simulink model "MainDrive_Kuehlung_V3_D"  (Simulink 7.6)
settings: Solver=ode45  StartTime=0.0  StopTime=SimulTime  RelTol=1e-3
values from neighbouring files (symbols this model uses):
  n = 0.8    [ParamtersSpindel_D.m]    (also in PlottingSpindel_Kuehlung_D.m = Scp_MainDrive.signals(4).values(:,1))
  n1 = 0.78    [ParamtersSpindel_D.m]
  n2 = 0.7    [ParamtersSpindel_D.m]
  p = 500    [ParamtersSpindel_D.m]
  p1 = 380    [ParamtersSpindel_D.m]
  p2 = 1100    [ParamtersSpindel_D.m]
  R = 25    [ParamtersSpindel_D.m]    (also in PlottingSpindel_Kuehlung_D.m = Scp_MainDriveT.signals(3).values(:,1)/1000)
  sb = 5.67*(10^-8)    (= 5.67e-08)    [ParamtersSpindel_D.m]
  T_amb = 290    [ParamtersSpindel_D.m]
  Venti_n2 = 273+40    (= 313)    [ParamtersSpindel_D.m]
undefined symbols (not defined in the file or in its folder): Job, magnitude, MainDrive, MainDriveCooling
libraries: simulink x1
settings Model: Creator=Coni  LastModifiedBy=conid

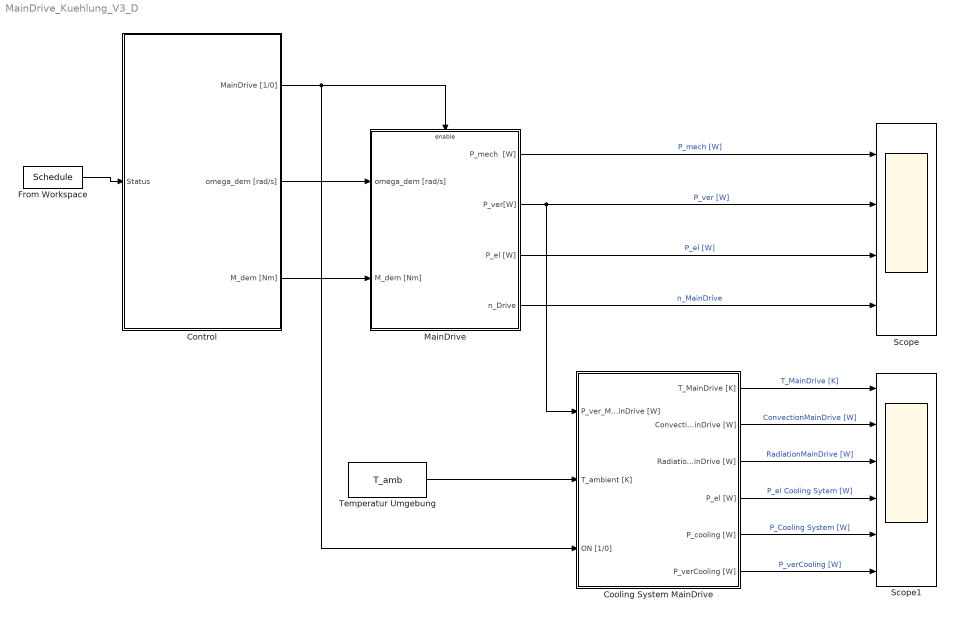
== system MainDrive_Kuehlung_V3_D ==
  Control : Subsystem  TreatAsAtomicUnit=on  mask{MainDrive=[0 1 1 1 1], Job=Job}
      mask prompts: Job "Job Struct"
      mask help:
      | Controls the components of the machine:
      |
      | Status:
      |     0. Off
      |     1. Standby
      |     2. Warmup
      |     3. Setting
      |     4. Machining
      |
      | If the status is machining, the job defined as
      |     - Job.time
      |     - Job.omega_dem
      |     - Job.M_dem
      | will be runned, and repeated.
      mask TabNameString: Status,Job
  Cooling System MainDrive : Subsystem  TreatAsAtomicUnit=on
  From Workspace : FromWorkspace  VariableName=Schedule  SampleTime=0  Interpolate=off  OutputAfterFinalValue=Holding final value
  MainDrive : Subsystem  TreatAsAtomicUnit=on
  Scope : Scope  NumInputPorts=4
      settings: TickLabels=on  TimeRange=100  YMin=0~-6e-010~-6e-010~-1.16573e-016  YMax=7e-026~-0~-0~-1.05471e-016  SaveName=Scp_MainDrive
  Scope1 : Scope  NumInputPorts=6
      settings: TickLabels=on  TimeRange=100  YMin=0~-5000~-2000~-0.1~-5~-5  YMax=16000~30000~14000~0.9~5~5  SaveName=Scp_MainDriveT
  Temperatur Umgebung : Constant  Value=T_amb
  wires:
  MainDrive/1(P_mech  [W]) -> Scope/1  "P_mech [W]"
  MainDrive/2(P_ver[W]) -> Scope/2, Cooling System MainDrive/1(P_ver_MainDrive [W])  "P_ver [W]"
  MainDrive/4(n_Drive) -> Scope/4  "n_MainDrive"
  Temperatur Umgebung/1 -> Cooling System MainDrive/2(T_ambient [K])
  MainDrive/3(P_el [W]) -> Scope/3  "P_el [W]"
  Cooling System MainDrive/1(T_MainDrive [K]) -> Scope1/1  "T_MainDrive [K]"
  Cooling System MainDrive/2(ConvectionMainDrive [W]) -> Scope1/2  "ConvectionMainDrive [W]"
  Cooling System MainDrive/3(RadiationMainDrive [W]) -> Scope1/3  "RadiationMainDrive [W]"
  Cooling System MainDrive/4(P_el [W]) -> Scope1/4  "P_el Cooling Sytem [W]"
  Cooling System MainDrive/5(P_cooling [W]) -> Scope1/5  "P_Cooling System [W]"
  Control/3(M_dem [Nm]) -> MainDrive/2(M_dem [Nm])
  From Workspace/1 -> Control/1(Status)
  Control/2(omega_dem [rad/s]) -> MainDrive/1(omega_dem [rad/s])
  Control/1(MainDrive [1/0]) -> MainDrive/Enable, Cooling System MainDrive/3(ON [1/0])
  Cooling System MainDrive/6(P_verCooling [W]) -> Scope1/6  "P_verCooling [W]"

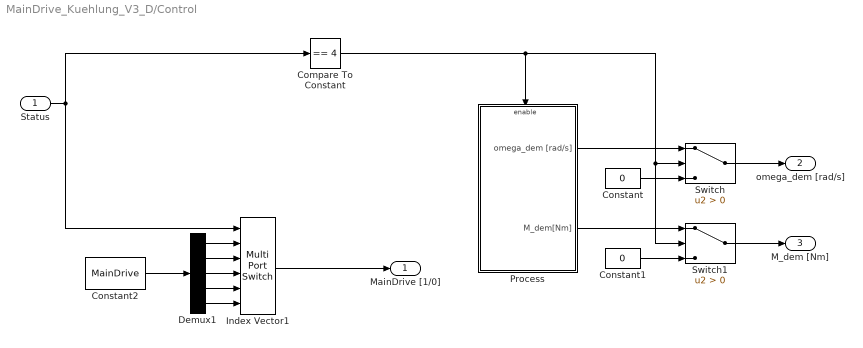
== system MainDrive_Kuehlung_V3_D/Control ==
  Status : Inport
  Compare To Constant : simulink/Logic and Bit Operations/Compare To Constant  SystemSampleTime=-1  relop===  const=4  LogicOutDataTypeMode=uint8
  Constant : Constant  Value=0
  Constant1 : Constant  Value=0
  Constant2 : Constant  Value=MainDrive
  Demux1 : Demux  Outputs=5
  Index Vector1 : MultiPortSwitch  DataPortOrder=Zero-based contiguous  Inputs=5  zeroidx=on
  Process : Subsystem  TreatAsAtomicUnit=on
  Switch : Switch  Criteria=u2 > Threshold
  Switch1 : Switch  Criteria=u2 > Threshold
  MainDrive [1/0] : Outport
  omega_dem [rad/s] : Outport  Port=2
  M_dem [Nm] : Outport  Port=3
  wires:
  Status/1 -> Compare To Constant/1, Index Vector1/1
  Demux1/1 -> Index Vector1/2
  Demux1/2 -> Index Vector1/3
  Demux1/3 -> Index Vector1/4
  Demux1/4 -> Index Vector1/5
  Demux1/5 -> Index Vector1/6
  Index Vector1/1 -> MainDrive [1/0]/1
  Compare To Constant/1 -> Process/Enable, Switch1/2, Switch/2
  Process/1(omega_dem [rad/s]) -> Switch/1
  Constant/1 -> Switch/3
  Process/2(M_dem[Nm]) -> Switch1/1
  Constant1/1 -> Switch1/3
  Switch/1 -> omega_dem [rad/s]/1
  Switch1/1 -> M_dem [Nm]/1
  Constant2/1 -> Demux1/1

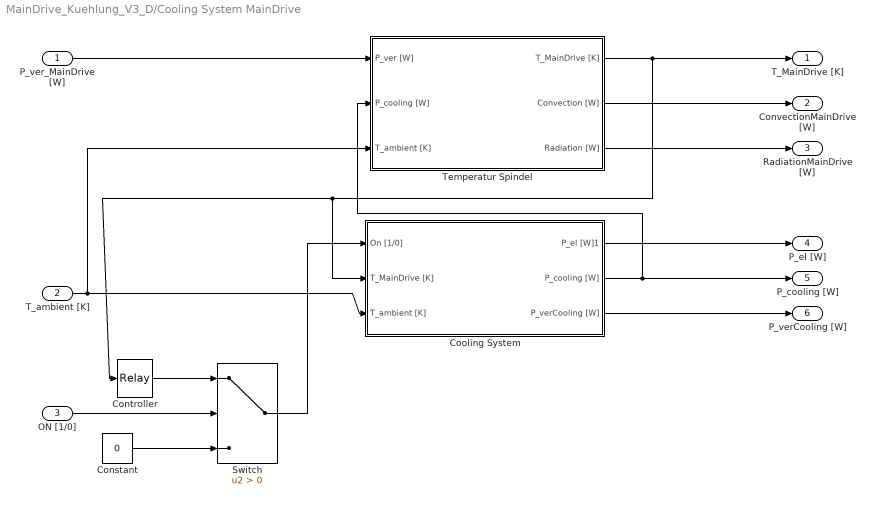
== system MainDrive_Kuehlung_V3_D/Cooling System MainDrive ==
  P_ver_MainDrive [W] : Inport
  T_ambient [K] : Inport  Port=2
  ON [1/0] : Inport  Port=3
  Constant : Constant  Value=0
  Controller : Relay  OnSwitchValue=MainDriveCooling.Tmax  OffSwitchValue=MainDriveCooling.Tmin
  Cooling System : Subsystem
  Switch : Switch  Criteria=u2 > Threshold
  Temperatur Spindel : Subsystem
  T_MainDrive [K] : Outport
  ConvectionMainDrive [W] : Outport  Port=2
  RadiationMainDrive [W] : Outport  Port=3
  P_el [W] : Outport  Port=4
  P_cooling [W] : Outport  Port=5
  P_verCooling [W] : Outport  Port=6
  wires:
  P_ver_MainDrive [W]/1 -> Temperatur Spindel/1(P_ver [W])
  Constant/1 -> Switch/3
  ON [1/0]/1 -> Switch/2
  Controller/1 -> Switch/1
  Temperatur Spindel/1(T_MainDrive [K]) -> Controller/1, Cooling System/2(T_MainDrive [K]), T_MainDrive [K]/1
  Switch/1 -> Cooling System/1(On [1/0])
  T_ambient [K]/1 -> Cooling System/3(T_ambient [K]), Temperatur Spindel/3(T_ambient [K])
  Temperatur Spindel/2(Convection [W]) -> ConvectionMainDrive [W]/1
  Temperatur Spindel/3(Radiation [W]) -> RadiationMainDrive [W]/1
  Cooling System/3(P_verCooling [W]) -> P_verCooling [W]/1
  Cooling System/1(P_el [W]1) -> P_el [W]/1
  Cooling System/2(P_cooling [W]) -> P_cooling [W]/1, Temperatur Spindel/2(P_cooling [W])

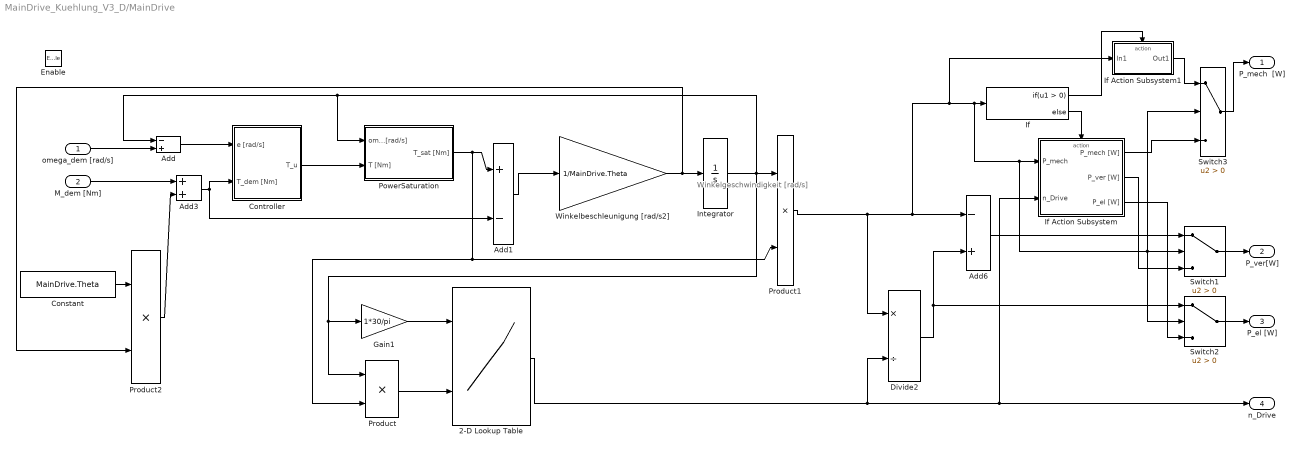
== system MainDrive_Kuehlung_V3_D/MainDrive ==
  note: Winkelgeschwindigkeit [rad/s]
  omega_dem [rad/s] : Inport
  M_dem [Nm] : Inport  Port=2
  Enable : EnablePort
  2-D Lookup Table : Lookup_n-D  BreakpointsForDimension1=MainDrive.Tabelomega  BreakpointsForDimension2=MainDrive.TabelM  Table=MainDrive.Tabeleta  InterpMethod=Cubic spline  ExtrapMethod=None - Clip  RndMeth=Simplest  InputSameDT=on
  Add : Sum  Inputs=-+
  Add1 : Sum  Inputs=+-
  Add3 : Sum
  Add6 : Sum  Inputs=-+
  Constant : Constant  Value=MainDrive.Theta
  Controller : Subsystem  TreatAsAtomicUnit=on
  Divide2 : Product  Inputs=*/
  Gain1 : Gain  Gain=1*30/pi
  If : If
  If Action Subsystem : Subsystem  TreatAsAtomicUnit=on
  If Action Subsystem1 : Subsystem  TreatAsAtomicUnit=on
  Integrator : Integrator
  PowerSaturation : Subsystem  TreatAsAtomicUnit=on
  Product : Product  RndMeth=Zero
  Product1 : Product  RndMeth=Zero
  Product2 : Product  RndMeth=Zero
  Switch1 : Switch  Criteria=u2 > Threshold
  Switch2 : Switch  Criteria=u2 > Threshold
  Switch3 : Switch  Criteria=u2 > Threshold
  Winkelbeschleunigung [rad/s2] : Gain  Gain=1/MainDrive.Theta
  P_mech  [W] : Outport
  P_ver[W] : Outport  Port=2
  P_el [W] : Outport  Port=3
  n_Drive : Outport  Port=4
  wires:
  omega_dem [rad/s]/1 -> Add/2
  Add/1 -> Controller/1(e [rad/s])
  Controller/1(T_u) -> PowerSaturation/2(T [Nm])
  PowerSaturation/1(T_sat [Nm]) -> Add1/1, Product1/2, Product/2
  Add1/1 -> Winkelbeschleunigung [rad/s2]/1
  Winkelbeschleunigung [rad/s2]/1 -> Integrator/1, Product2/2
  Integrator/1 -> Product1/1, Add/1, PowerSaturation/1(omega [rad/s]), Product/1, Gain1/1
  Product/1 -> 2-D Lookup Table/2
  Gain1/1 -> 2-D Lookup Table/1
  Constant/1 -> Product2/1
  Add3/1 -> Controller/2(T_dem [Nm]), Add1/2
  M_dem [Nm]/1 -> Add3/1
  Product2/1 -> Add3/2
  Product1/1 -> Add6/1, If/1, If Action Subsystem/1(P_mech), Switch1/2, Switch2/2, Switch3/2, If Action Subsystem1/1(In1), Divide2/1
  Divide2/1 -> Add6/2, Switch2/1
  2-D Lookup Table/1 -> n_Drive/1, If Action Subsystem/2(n_Drive), Divide2/2
  If/2 -> If Action Subsystem/Action
  Switch1/1 -> P_ver[W]/1
  Add6/1 -> Switch1/1
  If Action Subsystem/2(P_ver [W]) -> Switch1/3
  Switch2/1 -> P_el [W]/1
  If Action Subsystem/3(P_el [W]) -> Switch2/3
  If/1 -> If Action Subsystem1/Action
  If Action Subsystem1/1(Out1) -> Switch3/1
  Switch3/1 -> P_mech  [W]/1
  If Action Subsystem/1(P_mech [W]) -> Switch3/3

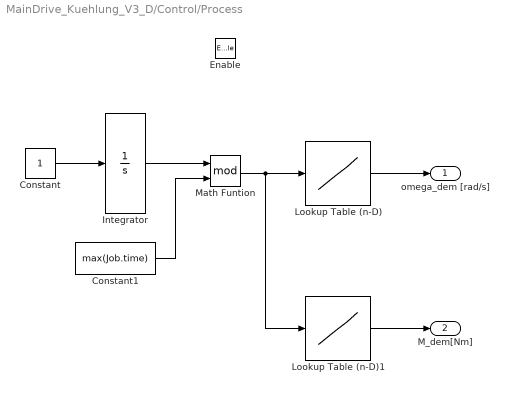
== system MainDrive_Kuehlung_V3_D/Control/Process ==
  Enable : EnablePort
  Constant : Constant
  Constant1 : Constant  Value=max(Job.time)
  Integrator : Integrator
  Lookup Table (n-D) : Lookup_n-D  NumberOfTableDimensions=1  BreakpointsForDimension1=Job.time  Table=Job.omega_dem  InterpMethod=None - Flat  ExtrapMethod=Cubic spline  InputSameDT=on
  Lookup Table (n-D)1 : Lookup_n-D  NumberOfTableDimensions=1  BreakpointsForDimension1=Job.time  Table=Job.M_dem  InterpMethod=None - Flat  InputSameDT=on
  Math Funtion : Math  Operator=mod  SaturateOnIntegerOverflow=on
  omega_dem [rad/s] : Outport
  M_dem[Nm] : Outport  Port=2
  wires:
  Constant/1 -> Integrator/1
  Integrator/1 -> Math Funtion/1
  Math Funtion/1 -> Lookup Table (n-D)/1, Lookup Table (n-D)1/1
  Lookup Table (n-D)/1 -> omega_dem [rad/s]/1
  Lookup Table (n-D)1/1 -> M_dem[Nm]/1
  Constant1/1 -> Math Funtion/2

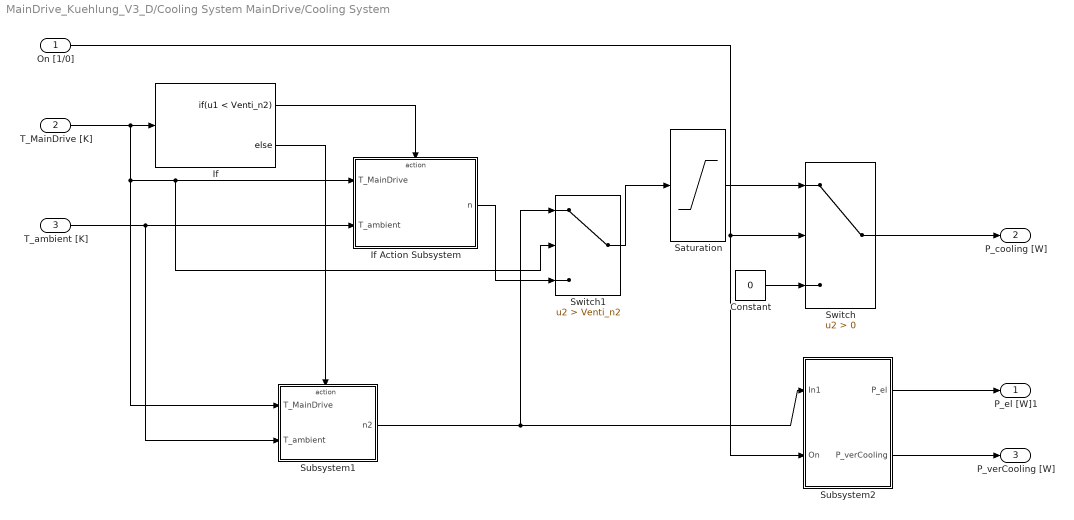
== system MainDrive_Kuehlung_V3_D/Cooling System MainDrive/Cooling System ==
  On [1/0] : Inport
  T_MainDrive [K] : Inport  Port=2
  T_ambient [K] : Inport  Port=3
  Constant : Constant  Value=0
  If : If  IfExpression=u1 < Venti_n2
  If Action Subsystem : Subsystem  TreatAsAtomicUnit=on
  Saturation : Saturate  UpperLimit=12000  LowerLimit=0
  Subsystem1 : Subsystem
  Subsystem2 : Subsystem
  Switch : Switch  Criteria=u2 > Threshold
  Switch1 : Switch  Criteria=u2 > Threshold  Threshold=Venti_n2
  P_el [W]1 : Outport
  P_cooling [W] : Outport  Port=2
  P_verCooling [W] : Outport  Port=3
  wires:
  T_ambient [K]/1 -> Subsystem1/2(T_ambient), If Action Subsystem/2(T_ambient)
  Constant/1 -> Switch/3
  On [1/0]/1 -> Switch/2, Subsystem2/2(On)
  Saturation/1 -> Switch/1
  Switch/1 -> P_cooling [W]/1
  T_MainDrive [K]/1 -> Subsystem1/1(T_MainDrive), If Action Subsystem/1(T_MainDrive), Switch1/2, If/1
  Subsystem1/1(n2) -> Switch1/1, Subsystem2/1(In1)
  Switch1/1 -> Saturation/1
  If/1 -> If Action Subsystem/Action
  If/2 -> Subsystem1/Action
  If Action Subsystem/1(n) -> Switch1/3
  Subsystem2/1(P_el) -> P_el [W]1/1
  Subsystem2/2(P_verCooling) -> P_verCooling [W]/1

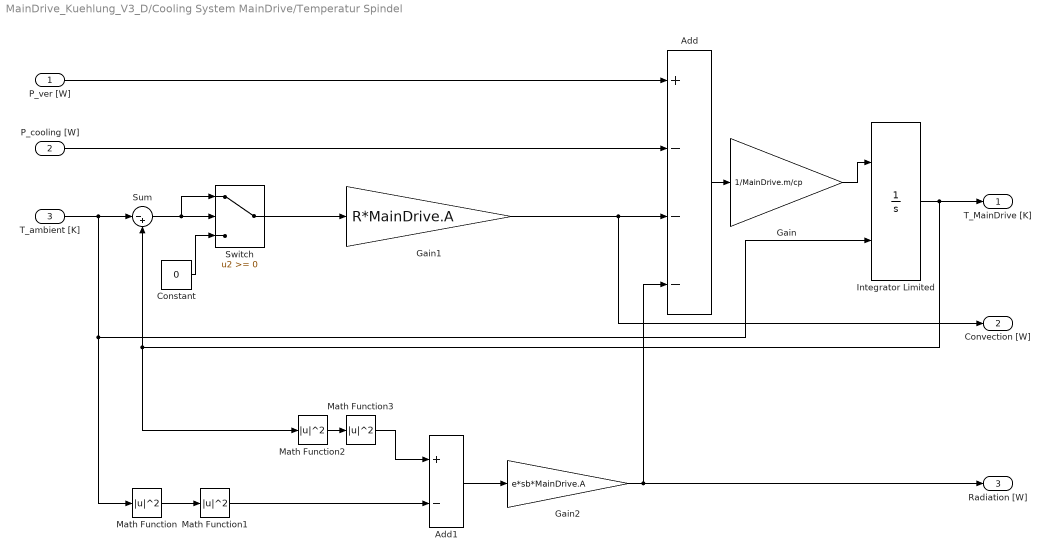
== system MainDrive_Kuehlung_V3_D/Cooling System MainDrive/Temperatur Spindel ==
  P_ver [W] : Inport
  P_cooling [W] : Inport  Port=2
  T_ambient [K] : Inport  Port=3
  Add : Sum  Inputs=+---
  Add1 : Sum  Inputs=+-
  Constant : Constant  Value=0
  Gain : Gain  Gain=1/MainDrive.m/cp
  Gain1 : Gain  Gain=R*MainDrive.A
  Gain2 : Gain  Gain=e*sb*MainDrive.A
  Integrator Limited : Integrator  InitialConditionSource=external  LimitOutput=on
  Math Function{,1..3} (4 alike) : Math  Operator=magnitude^2  SaturateOnIntegerOverflow=on
  Sum : Sum  Inputs=|-+
  Switch : Switch
  T_MainDrive [K] : Outport
  Convection [W] : Outport  Port=2
  Radiation [W] : Outport  Port=3
  wires:
  P_ver [W]/1 -> Add/1
  Gain/1 -> Integrator Limited/1
  Gain1/1 -> Convection [W]/1, Add/3
  Integrator Limited/1 -> T_MainDrive [K]/1, Sum/2, Math Function2/1
  Add/1 -> Gain/1
  Math Function/1 -> Math Function1/1
  Gain2/1 -> Radiation [W]/1, Add/4
  P_cooling [W]/1 -> Add/2
  T_ambient [K]/1 -> Sum/1, Integrator Limited/2, Math Function/1
  Sum/1 -> Switch/2, Switch/1
  Constant/1 -> Switch/3
  Math Function2/1 -> Math Function3/1
  Add1/1 -> Gain2/1
  Math Function3/1 -> Add1/1
  Math Function1/1 -> Add1/2
  Switch/1 -> Gain1/1

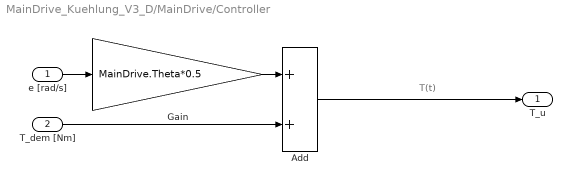
== system MainDrive_Kuehlung_V3_D/MainDrive/Controller ==
  note: T(t)
  e [rad/s] : Inport
  T_dem [Nm] : Inport  Port=2
  Add : Sum
  Gain : Gain  Gain=MainDrive.Theta*0.5
  T_u : Outport
  wires:
  Add/1 -> T_u/1
  T_dem [Nm]/1 -> Add/2
  Gain/1 -> Add/1
  e [rad/s]/1 -> Gain/1

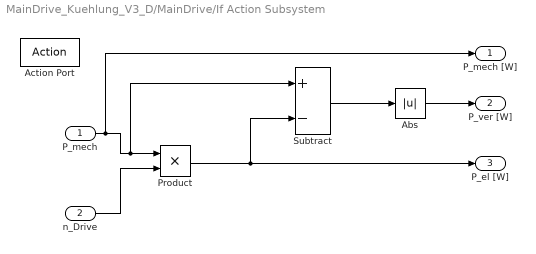
== system MainDrive_Kuehlung_V3_D/MainDrive/If Action Subsystem ==
  P_mech : Inport
  n_Drive : Inport  Port=2
  Action Port : ActionPort  ActionType=else
  Abs : Abs
  Product : Product  RndMeth=Zero
  Subtract : Sum  Inputs=+-
  P_mech [W] : Outport
  P_ver [W] : Outport  Port=2
  P_el [W] : Outport  Port=3
  wires:
  P_mech/1 -> Product/1, Subtract/1, P_mech [W]/1
  n_Drive/1 -> Product/2
  Product/1 -> P_el [W]/1, Subtract/2
  Abs/1 -> P_ver [W]/1
  Subtract/1 -> Abs/1

== system MainDrive_Kuehlung_V3_D/MainDrive/If Action Subsystem1 ==
  In1 : Inport
  Action Port : ActionPort  ActionType=then
  Out1 : Outport
  wires:
  In1/1 -> Out1/1

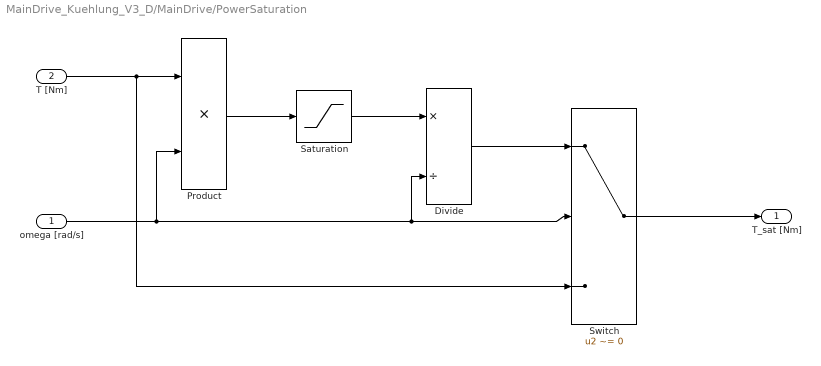
== system MainDrive_Kuehlung_V3_D/MainDrive/PowerSaturation ==
  omega [rad/s] : Inport
  T [Nm] : Inport  Port=2
  Divide : Product  Inputs=*/
  Product : Product  RndMeth=Zero
  Saturation : Saturate  UpperLimit=MainDrive.Pmax  LowerLimit=-MainDrive.Pmax
  Switch : Switch  Criteria=u2 ~= 0
  T_sat [Nm] : Outport
  wires:
  Product/1 -> Saturation/1
  Saturation/1 -> Divide/1
  Divide/1 -> Switch/1
  Switch/1 -> T_sat [Nm]/1
  T [Nm]/1 -> Product/1, Switch/3
  omega [rad/s]/1 -> Switch/2, Divide/2, Product/2

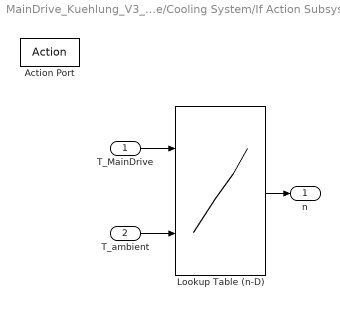
== system MainDrive_Kuehlung_V3_D/Cooling System MainDrive/Cooling System/If Action Subsystem ==
  T_MainDrive : Inport
  T_ambient : Inport  Port=2
  Action Port : ActionPort  ActionType=then
  Lookup Table (n-D) : Lookup_n-D  BreakpointsForDimension1=MainDriveCooling.Air.T_int  BreakpointsForDimension2=MainDriveCooling.Air.T_ext  Table=MainDriveCooling.Air.P  InterpMethod=Cubic spline  ExtrapMethod=None - Clip  InputSameDT=on
  n : Outport
  wires:
  T_ambient/1 -> Lookup Table (n-D)/2
  T_MainDrive/1 -> Lookup Table (n-D)/1
  Lookup Table (n-D)/1 -> n/1

== system MainDrive_Kuehlung_V3_D/Cooling System MainDrive/Cooling System/Subsystem1 ==
  T_MainDrive : Inport
  T_ambient : Inport  Port=2
  Action Port : ActionPort  ActionType=else
  Lookup Table (n-D)1 : Lookup_n-D  BreakpointsForDimension1=MainDriveCooling.Air.T_int  BreakpointsForDimension2=MainDriveCooling.Air.T_ext  Table=MainDriveCooling.Air.P_n2  InterpMethod=Cubic spline  ExtrapMethod=None - Clip  InputSameDT=on
  n2 : Outport
  wires:
  T_ambient/1 -> Lookup Table (n-D)1/2
  T_MainDrive/1 -> Lookup Table (n-D)1/1
  Lookup Table (n-D)1/1 -> n2/1

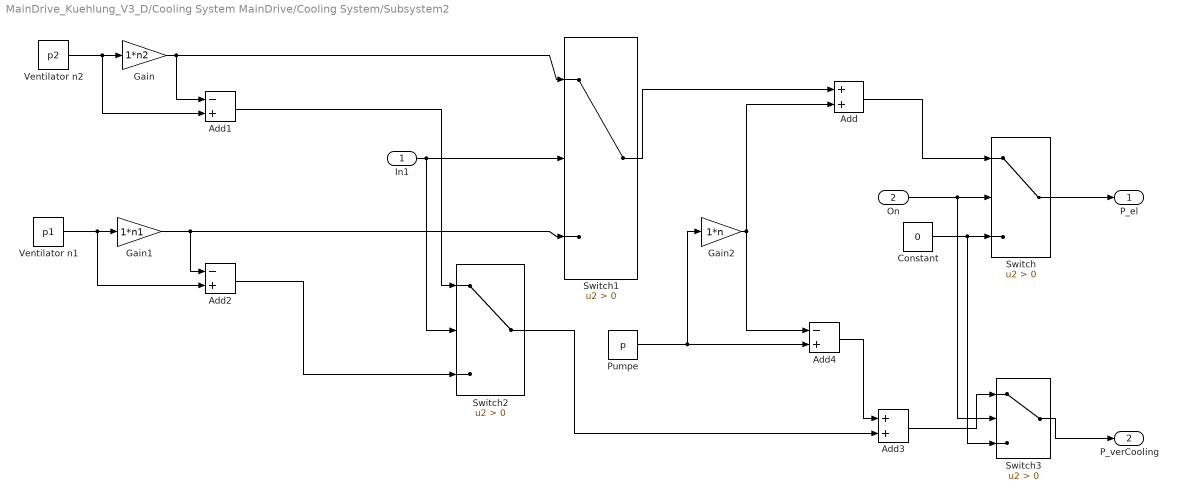
== system MainDrive_Kuehlung_V3_D/Cooling System MainDrive/Cooling System/Subsystem2 ==
  In1 : Inport
  On : Inport  Port=2
  Add : Sum
  Add1 : Sum  Inputs=-+
  Add2 : Sum  Inputs=-+
  Add3 : Sum
  Add4 : Sum  Inputs=-+
  Constant : Constant  Value=0
  Gain : Gain  Gain=1*n2
  Gain1 : Gain  Gain=1*n1
  Gain2 : Gain  Gain=1*n
  Pumpe : Constant  Value=p
  Switch{,1..3} (4 alike) : Switch  Criteria=u2 > Threshold
  Ventilator n1 : Constant  Value=p1
  Ventilator n2 : Constant  Value=p2
  P_el : Outport
  P_verCooling : Outport  Port=2
  wires:
  Switch1/1 -> Add/1
  In1/1 -> Switch1/2, Switch2/2
  Ventilator n2/1 -> Gain/1, Add1/2
  Gain/1 -> Switch1/1, Add1/1
  Gain1/1 -> Switch1/3, Add2/1
  Ventilator n1/1 -> Gain1/1, Add2/2
  Gain2/1 -> Add/2, Add4/1
  Pumpe/1 -> Gain2/1, Add4/2
  Add4/1 -> Add3/1
  Add1/1 -> Switch2/1
  Add2/1 -> Switch2/3
  Switch2/1 -> Add3/2
  On/1 -> Switch/2, Switch3/2
  Switch/1 -> P_el/1
  Add/1 -> Switch/1
  Constant/1 -> Switch/3, Switch3/3
  Switch3/1 -> P_verCooling/1
  Add3/1 -> Switch3/1
